simulink model "MainPendulum"  (R2025b)
settings: Solver=VariableStepAuto  StartTime=0.0  StopTime=20.0  RelTol=1e-3
values from neighbouring files (symbols this model uses):
  u0 = lin.u0    [linearize_nonlinear_plant.m]    (also in linearize_rotpendulum.m = settingOrDefault(settings, 'u0', 0); linearized_plant.mat = 0; linearized_plant_eq_pi_pi.mat = 0; rotpendulumEkfStateTransition.m = ekfInput(3))
  x0 = [theta_1_0; theta_2_0; theta_1_dot_0; theta_2_dot_0]    [build_sysid_parameters.m]    (also in linearize_nonlinear_plant.m = lin.x0; linearize_rotpendulum.m = x0(:); linearized_plant.mat = [3.14159265359 3.14159265359 0 0]; linearized_plant_eq_pi_pi.mat = [3.14159265359 3.14159265359 0 0])
settings Model: Creator=djangovanderplas  LastModifiedBy=thoma

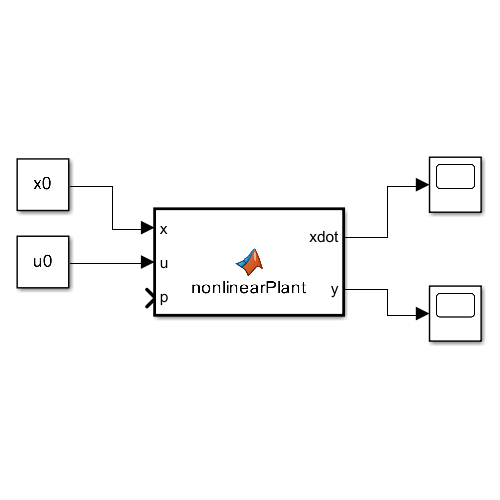
[thumbnail: Simulink's stored preview of the top-level diagram]
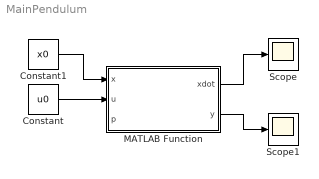
== system MainPendulum ==
  Constant : Constant  Value=u0
  Constant1 : Constant  Value=x0
  MATLAB Function : MATLAB Function  TreatAsAtomicUnit=on
  Scope : Scope
  Scope1 : Scope
  wires:
  Constant/1 -> MATLAB Function/2(u)
  Constant1/1 -> MATLAB Function/1(x)
  MATLAB Function/1(xdot) -> Scope/1
  MATLAB Function/2(y) -> Scope1/1

== matlab function MainPendulum/MATLAB Function ==
  data: xdot output; x input; y output; u input; p input
function [xdot, y] = nonlinearPlant(x, u, p)
%#codegen
% nonlinearPlant
%
% Reduced nonlinear plant model for the rotational double pendulum.
%
% Inputs:
%   x = [theta1; theta2; theta1_dot; theta2_dot]
%   u = motor input command / voltage-like input
%   p = parameter vector loaded from .mat file
%
% Outputs:
%   xdot = state derivative
%   y    = measured output [theta1; theta2]

% ------------------------------------------------------------
% 1. States
% ------------------------------------------------------------
theta1  = x(1);
theta2  = x(2);
dtheta1 = x(3);
dtheta2 = x(4);

% ------------------------------------------------------------
% 2. Unpack parameter vector
% ------------------------------------------------------------
pa       = p(1);

pb1      = p(2);
pc1      = p(3);
pg1      = p(4);
pu       = p(5);
p0       = p(6);

pb2      = p(7);
pg2      = p(8);
pc2      = p(9);
psdelta2 = p(10);
vs2      = p(11);

epsv1    = p(12);
epsv2    = p(13);

pc       = p(14);

% ------------------------------------------------------------
% 3. Inertia matrix M(q)
% ------------------------------------------------------------
c2 = cos(theta2);
s2 = sin(theta2);

M11 = pa + 1 + 2*pc*c2;
M12 = 1 + pc*c2;
M21 = M12;
M22 = 1;

% ------------------------------------------------------------
% 4. Coriolis/centrifugal term C(q,qdot)*qdot
% ------------------------------------------------------------
Cqdot1 = -pc*s2*(2*dtheta1*dtheta2 + dtheta2^2);
Cqdot2 =  pc*s2*dtheta1^2;

% ------------------------------------------------------------
% 5. Friction vector F(qdot)
% ------------------------------------------------------------
F1 = pb1*dtheta1 + pc1*tanh(dtheta1/epsv1);

stribeck2 = pc2 + psdelta2*exp(-(dtheta2/vs2)^2);
F2 = pb2*dtheta2 + stribeck2*tanh(dtheta2/epsv2);

% ------------------------------------------------------------
% 6. Gravity vector G(q)
% ------------------------------------------------------------
G1 = -pg1*sin(theta1) - pg2*sin(theta1 + theta2);
G2 = -pg2*sin(theta1 + theta2);

% ------------------------------------------------------------
% 7. Input vector I(V)
% ------------------------------------------------------------
I1 = pu*u + p0;
I2 = 0;

% ------------------------------------------------------------
% 8. Solve M(q)*qddot = I - Cqdot - F - G
% ------------------------------------------------------------
rhs1 = I1 - Cqdot1 - F1 - G1;
rhs2 = I2 - Cqdot2 - F2 - G2;

detM = M11*M22 - M12*M21;

ddtheta1 = ( M22*rhs1 - M12*rhs2) / detM;
ddtheta2 = (-M21*rhs1 + M11*rhs2) / detM;

% ------------------------------------------------------------
% 9. State derivative
% ------------------------------------------------------------
xdot = zeros(4,1);

xdot(1) = dtheta1;
xdot(2) = dtheta2;
xdot(3) = ddtheta1;
xdot(4) = ddtheta2;

% ------------------------------------------------------------
% 10. Outputs
% ------------------------------------------------------------
y = zeros(2,1);

y(1) = theta1;
y(2) = theta2;

end
